simulink model "CAMFC2_04_Quad_03_R2017b"  (R2017b)
settings: Solver=ode45  StartTime=0.0  StopTime=600  RelTol=1e-3  EnableMultiTasking=on
InitFcn:
  | constant_CAMFC2_04_Quad_03
values from neighbouring files (symbols this model uses):
  alpha = 0.1    [constant_CAMFC2_01_WMR01.m]    (also in constant_CAMFC2_04_Comp.m = 0.01; constant_CAMFC2_04_Quad_03.m; constant_CAMFC2_04_Simple.m = 0.01; constant_CAMFC2_04_Simple_DoubleIntegrator.m = 0.01)
  AN = [     0 1 0 0 ... (first row only)    [constant_CAMFC2_01_WMR01.m]    (also in constant_CAMFC2_04_Comp.m = [     0 1 0 0 1; constant_CAMFC2_04_Quad_03.m; constant_CAMFC2_04_Simple.m; constant_CAMFC2_04_Simple_DoubleIntegrator.m)
  B = eye(n)    [constant_CAMFC2_01_WMR01.m]    (also in constant_CAMFC2_04_Quad_03.m; constant_CAMFC2_Quad_New_02.m)
  BBT_inv = ((B'*B)^(-1))*B'    [constant_CAMFC2_04_Quad_03.m]    (also in constant_CAMFC2_Quad_New_02.m)
  Beta = 0.2    [constant_CAMFC2_04_Quad_03.m]    (also in constant_CAMFC2_Quad_New_02.m = 0.1)
  BN = [     1 0 0 0 ... (first row only)    [constant_CAMFC2_01_WMR01.m]    (also in constant_CAMFC2_04_Comp.m = [     0 0 0 0 0; constant_CAMFC2_04_Quad_03.m; constant_CAMFC2_04_Simple.m; constant_CAMFC2_04_Simple_DoubleIntegrator.m)
  Bv = eye(n0)    [constant_CAMFC2_04_Quad_03.m]
  BvBT_inv = ((Bv'*Bv)^(-1))*Bv'    [constant_CAMFC2_04_Quad_03.m]
  chi = [0 0 0 0 ... (first row only)    [constant_CAMFC2_01_WMR01.m]    (also in constant_CAMFC2_04_Comp.m = X_m*ones(n0,1); constant_CAMFC2_04_Quad_03.m = X_m*ones(n0,1); constant_CAMFC2_04_Simple.m = X_m*ones(n0,1); constant_CAMFC2_04_Simple_DoubleIntegrator.m = X_m*ones(n0,1))
  epsilon_struct = struct('data',epsilon_InitVal)    [constant_CAMFC2_01_WMR01.m]    (also in constant_CAMFC2_04_Comp.m; constant_CAMFC2_04_Quad_03.m; constant_CAMFC2_04_Simple.m; constant_CAMFC2_04_Simple_DoubleIntegrator.m)
  gama1 = 1e4*diag([1e-6*ones(2,1);1e0*ones(2,1)])    [constant_CAMFC2_01_WMR01.m]    (also in constant_CAMFC2_04_Comp.m = 1e+3*diag([1e-6;1e-0]); constant_CAMFC2_04_Quad_03.m = 1e+2*diag(1e-0*ones(n0,1)); constant_CAMFC2_04_Simple.m = 1e+2*diag([1e-0;1e-0]); constant_CAMFC2_04_Simple_Formation.m = 1e+2*diag([1e-0;1e-0]))
  gama2 = 1e-2*diag([1e-6*ones(2,1);1e0*ones(2,1)])    [constant_CAMFC2_01_WMR01.m]    (also in constant_CAMFC2_04_Comp.m = 1e+0*diag([1e-6;1e-0]); constant_CAMFC2_04_Quad_03.m = 1e+0*diag(1e-0*ones(n0,1)); constant_CAMFC2_04_Simple.m = 1e+1*diag([1e-0;1e-0]); constant_CAMFC2_04_Simple_Formation.m = 1e+1*diag([1e-0;1e-0]))
  gamma_0 = 1e+0*diag([1e-0*ones(n0,1);1e-0*ones(n0,1)])    [constant_CAMFC2_04_Quad_03.m]    (also in constant_CAMFC2_Quad_New_02.m = 1e-2*diag([1e-6*ones(n0,1);1e-0*ones(n0,1)]))
  gamma_0v = 1e-0*diag(1e-0*ones(n0,1))    [constant_CAMFC2_04_Quad_03.m]
  gamma_1 = 1e+2*diag([1e-0*ones(n0,1);1e-0*ones(n0,1)])    [constant_CAMFC2_04_Quad_03.m]    (also in constant_CAMFC2_Quad_New_02.m = 1e+1*diag([1e-6*ones(n0,1);1e-0*ones(n0,1)]))
  gamma_1v = 1e+2*diag(1e-0*ones(n0,1))    [constant_CAMFC2_04_Quad_03.m]
  ge = 9.81    [constant_CAMFC2_04_Comp.m]    (also in constant_CAMFC2_04_Quad_03.m; constant_CAMFC2_04_Simple.m; constant_CAMFC2_04_Simple_DoubleIntegrator.m; constant_CAMFC2_04_Simple_DoubleIntegrator_02.m)
  H = L + BN    [constant_CAMFC2_01_WMR01.m]    (also in constant_CAMFC2_04_Comp.m; constant_CAMFC2_04_Quad_03.m; constant_CAMFC2_04_Simple.m; constant_CAMFC2_04_Simple_DoubleIntegrator.m)
  J = 0.01    [constant_CAMFC2_01_WMR01.m]    (also in constant_CAMFC2_04_Quad_03.m = 1.0e-3 * diag([1 1 2],0); constant_CAMFC2_Quad_New_02.m = 1.2416e-3 * diag([1 1 2],0))
  k1 = 1    [constant_CAMFC2_01_WMR01.m]    (also in constant_CAMFC2_04_Comp.m; constant_CAMFC2_04_Quad_03.m = 50; constant_CAMFC2_04_Simple.m; constant_CAMFC2_04_Simple_DoubleIntegrator.m)
  k2 = 1    [constant_CAMFC2_01_WMR01.m]    (also in constant_CAMFC2_04_Comp.m; constant_CAMFC2_04_Quad_03.m; constant_CAMFC2_04_Simple.m; constant_CAMFC2_04_Simple_DoubleIntegrator.m)
  Ka = 0.1    [constant_CAMFC2_04_Quad_03.m]    (also in constant_CAMFC2_Quad_New_02.m = 0.01)
  Kd = 0.1    [constant_CAMFC2_04_Quad_03.m]    (also in constant_CAMFC2_Quad_New_02.m = 0.01)
  m = 6    [constant_CAMFC2_04_Quad_03.m]    (also in constant_CAMFC2_Quad_New_02.m)
  M = 1    [constant_CAMFC2_01_WMR01.m]    (also in constant_CAMFC2_04_Quad_03.m = 2; constant_CAMFC2_Quad_New_02.m = 2)
  N = 4    [constant_CAMFC2_01_WMR01.m]    (also in constant_CAMFC2_04_Comp.m = 5; constant_CAMFC2_04_Quad_03.m; constant_CAMFC2_04_Simple.m; constant_CAMFC2_04_Simple_DoubleIntegrator.m)
  n = 4    [constant_CAMFC2_01_WMR01.m]    (also in constant_CAMFC2_04_Comp.m = 2; constant_CAMFC2_04_Quad_03.m = 6; constant_CAMFC2_04_Simple.m = 2; constant_CAMFC2_04_Simple_DoubleIntegrator.m = 2)
  n0 = 2    [constant_CAMFC2_01_WMR01.m]    (also in constant_CAMFC2_04_Comp.m = 1; constant_CAMFC2_04_Quad_03.m = 3; constant_CAMFC2_04_Simple.m; constant_CAMFC2_04_Simple_DoubleIntegrator.m = 1)
  noise_amp = 0.1    [constant_CAMFC2_04_Quad_03.m]
  noise_frq = 1    [constant_CAMFC2_04_Quad_03.m]
  Observer_Gain = 100    [constant_CAMFC2_01_WMR01.m]    (also in constant_CAMFC2_04_Comp.m = 10; constant_CAMFC2_04_Quad_03.m = 1; constant_CAMFC2_04_Simple.m; constant_CAMFC2_04_Simple_DoubleIntegrator.m)
  Observer_Gain1 = 100    [constant_CAMFC2_01_WMR01.m]    (also in constant_CAMFC2_04_Comp.m = 10; constant_CAMFC2_04_Quad_03.m = 1; constant_CAMFC2_04_Simple.m; constant_CAMFC2_04_Simple_DoubleIntegrator.m)
  P_struct = struct('data',P_InitVal)    [constant_CAMFC2_01_WMR01.m]    (also in constant_CAMFC2_04_Comp.m; constant_CAMFC2_04_Quad_03.m; constant_CAMFC2_04_Simple.m; constant_CAMFC2_04_Simple_DoubleIntegrator.m)
  Q = 1e-0*eye(n)    [constant_CAMFC2_01_WMR01.m]    (also in constant_CAMFC2_04_Comp.m = 1.0e+2*eye(n); constant_CAMFC2_04_Quad_03.m = 1e-0*eye(n0); constant_CAMFC2_04_Simple.m = 1.0e+1*eye(n); constant_CAMFC2_04_Simple_Formation.m = 1.0e+1*eye(n))
  QR = 1e-0*eye(n)    [constant_CAMFC2_04_Quad_03.m]    (also in constant_CAMFC2_Quad_New_02.m = 1e+0*eye(n))
  Qv = 1e-0*eye(n0)    [constant_CAMFC2_04_Quad_03.m]
  R = 1e-0*eye(n)    [constant_CAMFC2_01_WMR01.m]    (also in constant_CAMFC2_04_Quad_03.m; constant_CAMFC2_Quad_New_02.m = 1e+0*eye(n))
  r_formX = 1.0    (= 1)    [constant_CAMFC2_04_Quad_03.m]    (also in constant_CAMFC2_Quad_New_02.m)
  r_formY = 1.0    (= 1)    [constant_CAMFC2_04_Quad_03.m]    (also in constant_CAMFC2_Quad_New_02.m)
  r_formZ = 0.5    [constant_CAMFC2_04_Quad_03.m]    (also in constant_CAMFC2_Quad_New_02.m = 1)
  rho1 = 1e-1    (= 0.1)    [constant_CAMFC2_01_WMR01.m]    (also in constant_CAMFC2_04_Comp.m = 1; constant_CAMFC2_04_Quad_03.m = 1; constant_CAMFC2_04_Simple.m = 1; constant_CAMFC2_04_Simple_DoubleIntegrator.m = 1)
  rho2 = 1e-3    (= 0.001)    [constant_CAMFC2_01_WMR01.m]    (also in constant_CAMFC2_04_Comp.m = 1; constant_CAMFC2_04_Quad_03.m = 1; constant_CAMFC2_04_Simple.m = 1; constant_CAMFC2_04_Simple_DoubleIntegrator.m = 10)
  rho_0 = 1e-0    (= 1)    [constant_CAMFC2_04_Quad_03.m]    (also in constant_CAMFC2_Quad_New_02.m = 0.01)
  rho_0v = 1e-0    (= 1)    [constant_CAMFC2_04_Quad_03.m]
  rho_1 = 1e-0    (= 1)    [constant_CAMFC2_04_Quad_03.m]    (also in constant_CAMFC2_Quad_New_02.m = 0.01)
  rho_1v = 1e-0    (= 1)    [constant_CAMFC2_04_Quad_03.m]
  Rv = 1e-0*eye(n0)    [constant_CAMFC2_04_Quad_03.m]
  T_struct = struct('data',T_InitVal)    [constant_CAMFC2_01_WMR01.m]    (also in constant_CAMFC2_04_Comp.m; constant_CAMFC2_04_Quad_03.m; constant_CAMFC2_04_Simple.m; constant_CAMFC2_04_Simple_DoubleIntegrator.m)
  Upsilon_M = Upsilon_m*ones(n,1)    [constant_CAMFC2_01_WMR01.m]    (also in constant_CAMFC2_04_Comp.m; constant_CAMFC2_04_Quad_03.m = Upsilon_m*ones(n0,1); constant_CAMFC2_04_Simple.m; constant_CAMFC2_04_Simple_DoubleIntegrator.m)
  Vel_limit = 100    [constant_CAMFC2_04_Quad_03.m]
(part 2 of 4)

== system CAMFC2_04_Quad_03_R2017b/Data Bus /Observers Log/For matrix Plot11 ==
  T : Inport
  MATLAB Function : MATLAB Function  TreatAsAtomicUnit=on
  To Workspace : ToWorkspace  VariableName=T4  SaveFormat=Structure With Time  SampleTime=-1
  wires:
  MATLAB Function/1(y) -> To Workspace/1
  T/1 -> MATLAB Function/1(u)

== system CAMFC2_04_Quad_03_R2017b/Data Bus /Observers Log/For matrix Plot12 ==
  epsilon : Inport
  MATLAB Function : MATLAB Function  TreatAsAtomicUnit=on
  To Workspace : ToWorkspace  VariableName=epsilon1  SaveFormat=Structure With Time  SampleTime=-1
  wires:
  epsilon/1 -> MATLAB Function/1(u)
  MATLAB Function/1(y) -> To Workspace/1

== system CAMFC2_04_Quad_03_R2017b/Data Bus /Observers Log/For matrix Plot13 ==
  epsilon : Inport
  MATLAB Function : MATLAB Function  TreatAsAtomicUnit=on
  To Workspace : ToWorkspace  VariableName=epsilon2  SaveFormat=Structure With Time  SampleTime=-1
  wires:
  MATLAB Function/1(y) -> To Workspace/1
  epsilon/1 -> MATLAB Function/1(u)

== system CAMFC2_04_Quad_03_R2017b/Data Bus /Observers Log/For matrix Plot14 ==
  epsilon : Inport
  MATLAB Function : MATLAB Function  TreatAsAtomicUnit=on
  To Workspace : ToWorkspace  VariableName=epsilon3  SaveFormat=Structure With Time  SampleTime=-1
  wires:
  MATLAB Function/1(y) -> To Workspace/1
  epsilon/1 -> MATLAB Function/1(u)

== system CAMFC2_04_Quad_03_R2017b/Data Bus /Observers Log/For matrix Plot15 ==
  epsilon : Inport
  MATLAB Function : MATLAB Function  TreatAsAtomicUnit=on
  To Workspace : ToWorkspace  VariableName=epsilon4  SaveFormat=Structure With Time  SampleTime=-1
  wires:
  epsilon/1 -> MATLAB Function/1(u)
  MATLAB Function/1(y) -> To Workspace/1

== system CAMFC2_04_Quad_03_R2017b/Data Bus /Observers Log/For matrix Plot8 ==
  T : Inport
  MATLAB Function : MATLAB Function  TreatAsAtomicUnit=on
  To Workspace : ToWorkspace  VariableName=T1  SaveFormat=Structure With Time  SampleTime=-1
  wires:
  MATLAB Function/1(y) -> To Workspace/1
  T/1 -> MATLAB Function/1(u)

== system CAMFC2_04_Quad_03_R2017b/Data Bus /Observers Log/For matrix Plot9 ==
  T : Inport
  MATLAB Function : MATLAB Function  TreatAsAtomicUnit=on
  To Workspace : ToWorkspace  VariableName=T2  SaveFormat=Structure With Time  SampleTime=-1
  wires:
  T/1 -> MATLAB Function/1(u)
  MATLAB Function/1(y) -> To Workspace/1

== system CAMFC2_04_Quad_03_R2017b/Data Bus /Reference Trajectory/Subsystem ==
  Clock1 : Clock
  Desired Position4 : Constant  Value=0  VectorParams1D=off
  From Workspace : FromWorkspace  VariableName=RECT_X  SampleTime=0
  From Workspace1 : FromWorkspace  VariableName=RECT_Y  SampleTime=0
  From Workspace3 : FromWorkspace  VariableName=RECT_Z  SampleTime=0
  Gain : Gain  Gain=1/5
  Gain1 : Gain  Gain=1/5
  Gain2 : Gain
  Scope2 : Scope  NumInputPorts=3
  Switch : Switch  Criteria=u2 > Threshold  Threshold=10
  Transfer Fcn1 : TransferFcn  Numerator=[Beta]  Denominator=[1 Beta]
  Transfer Fcn2 : TransferFcn  Numerator=[Beta]  Denominator=[1 Beta]
  Transfer Fcn3 : TransferFcn  Numerator=[Beta]  Denominator=[1 Beta]
  Xd : Outport
  Yd : Outport  Port=2
  Zd : Outport  Port=3
  wires:
  From Workspace/1 -> Gain/1
  From Workspace1/1 -> Gain1/1
  Clock1/1 -> Switch/2
  Switch/1 -> Transfer Fcn1/1
  From Workspace3/1 -> Gain2/1
  Desired Position4/1 -> Switch/3
  Transfer Fcn1/1 -> Zd/1, Scope2/3
  Transfer Fcn2/1 -> Yd/1, Scope2/2
  Transfer Fcn3/1 -> Xd/1, Scope2/1
  Gain/1 -> Transfer Fcn3/1
  Gain1/1 -> Transfer Fcn2/1
  Gain2/1 -> Switch/1

== system CAMFC2_04_Quad_03_R2017b/Data Bus /Rotational Log/For matrix Plot ==
  P : Inport
  MATLAB Function : MATLAB Function  TreatAsAtomicUnit=on
  To Workspace : ToWorkspace  VariableName=P1_R  SaveFormat=Structure With Time  SampleTime=-1
  wires:
  MATLAB Function/1(y) -> To Workspace/1
  P/1 -> MATLAB Function/1(u)

== system CAMFC2_04_Quad_03_R2017b/Data Bus /Rotational Log/For matrix Plot1 ==
  P : Inport
  MATLAB Function : MATLAB Function  TreatAsAtomicUnit=on
  To Workspace : ToWorkspace  VariableName=P2_R  SaveFormat=Structure With Time  SampleTime=-1
  wires:
  P/1 -> MATLAB Function/1(u)
  MATLAB Function/1(y) -> To Workspace/1

== system CAMFC2_04_Quad_03_R2017b/Data Bus /Rotational Log/For matrix Plot2 ==
  P : Inport
  MATLAB Function : MATLAB Function  TreatAsAtomicUnit=on
  To Workspace : ToWorkspace  VariableName=P3_R  SaveFormat=Structure With Time  SampleTime=-1
  wires:
  P/1 -> MATLAB Function/1(u)
  MATLAB Function/1(y) -> To Workspace/1

== system CAMFC2_04_Quad_03_R2017b/Data Bus /Rotational Log/For matrix Plot3 ==
  P : Inport
  MATLAB Function : MATLAB Function  TreatAsAtomicUnit=on
  To Workspace : ToWorkspace  VariableName=P4_R  SaveFormat=Structure With Time  SampleTime=-1
  wires:
  MATLAB Function/1(y) -> To Workspace/1
  P/1 -> MATLAB Function/1(u)

== system CAMFC2_04_Quad_03_R2017b/Data Bus /Rotational Log/For matrix Plot4 ==
  A_hat : Inport
  MATLAB Function : MATLAB Function  TreatAsAtomicUnit=on
  To Workspace : ToWorkspace  VariableName=A_hat1_R  SaveFormat=Structure With Time  SampleTime=-1
  wires:
  A_hat/1 -> MATLAB Function/1(u)
  MATLAB Function/1(y) -> To Workspace/1

== system CAMFC2_04_Quad_03_R2017b/Data Bus /Rotational Log/For matrix Plot5 ==
  A_hat : Inport
  MATLAB Function : MATLAB Function  TreatAsAtomicUnit=on
  To Workspace : ToWorkspace  VariableName=A_hat2_R  SaveFormat=Structure With Time  SampleTime=-1
  wires:
  MATLAB Function/1(y) -> To Workspace/1
  A_hat/1 -> MATLAB Function/1(u)

== system CAMFC2_04_Quad_03_R2017b/Data Bus /Rotational Log/For matrix Plot6 ==
  A_hat : Inport
  MATLAB Function : MATLAB Function  TreatAsAtomicUnit=on
  To Workspace : ToWorkspace  VariableName=A_hat3_R  SaveFormat=Structure With Time  SampleTime=-1
  wires:
  A_hat/1 -> MATLAB Function/1(u)
  MATLAB Function/1(y) -> To Workspace/1

== system CAMFC2_04_Quad_03_R2017b/Data Bus /Rotational Log/For matrix Plot7 ==
  A_hat : Inport
  MATLAB Function : MATLAB Function  TreatAsAtomicUnit=on
  To Workspace : ToWorkspace  VariableName=A_hat4_R  SaveFormat=Structure With Time  SampleTime=-1
  wires:
  MATLAB Function/1(y) -> To Workspace/1
  A_hat/1 -> MATLAB Function/1(u)

== system CAMFC2_04_Quad_03_R2017b/Data Bus /Translational Log/For matrix Plot ==
  P : Inport
  MATLAB Function : MATLAB Function  TreatAsAtomicUnit=on
  To Workspace : ToWorkspace  VariableName=P1_TP  SaveFormat=Structure With Time  SampleTime=-1
  wires:
  P/1 -> MATLAB Function/1(u)
  MATLAB Function/1(y) -> To Workspace/1

== system CAMFC2_04_Quad_03_R2017b/Data Bus /Translational Log/For matrix Plot1 ==
  P : Inport
  MATLAB Function : MATLAB Function  TreatAsAtomicUnit=on
  To Workspace : ToWorkspace  VariableName=P2_TP  SaveFormat=Structure With Time  SampleTime=-1
  wires:
  MATLAB Function/1(y) -> To Workspace/1
  P/1 -> MATLAB Function/1(u)

== system CAMFC2_04_Quad_03_R2017b/Data Bus /Translational Log/For matrix Plot2 ==
  P : Inport
  MATLAB Function : MATLAB Function  TreatAsAtomicUnit=on
  To Workspace : ToWorkspace  VariableName=P3_TP  SaveFormat=Structure With Time  SampleTime=-1
  wires:
  MATLAB Function/1(y) -> To Workspace/1
  P/1 -> MATLAB Function/1(u)

== system CAMFC2_04_Quad_03_R2017b/Data Bus /Translational Log/For matrix Plot3 ==
  P : Inport
  MATLAB Function : MATLAB Function  TreatAsAtomicUnit=on
  To Workspace : ToWorkspace  VariableName=P4_TP  SaveFormat=Structure With Time  SampleTime=-1
  wires:
  P/1 -> MATLAB Function/1(u)
  MATLAB Function/1(y) -> To Workspace/1

== system CAMFC2_04_Quad_03_R2017b/Data Bus /Translational Log/For matrix Plot4 ==
  A_hat : Inport
  MATLAB Function : MATLAB Function  TreatAsAtomicUnit=on
  To Workspace : ToWorkspace  VariableName=A_hat1_TP  SaveFormat=Structure With Time  SampleTime=-1
  wires:
  MATLAB Function/1(y) -> To Workspace/1
  A_hat/1 -> MATLAB Function/1(u)

== system CAMFC2_04_Quad_03_R2017b/Data Bus /Translational Log/For matrix Plot5 ==
  A_hat : Inport
  MATLAB Function : MATLAB Function  TreatAsAtomicUnit=on
  To Workspace : ToWorkspace  VariableName=A_hat2_TP  SaveFormat=Structure With Time  SampleTime=-1
  wires:
  A_hat/1 -> MATLAB Function/1(u)
  MATLAB Function/1(y) -> To Workspace/1

== system CAMFC2_04_Quad_03_R2017b/Data Bus /Translational Log/For matrix Plot6 ==
  A_hat : Inport
  MATLAB Function : MATLAB Function  TreatAsAtomicUnit=on
  To Workspace : ToWorkspace  VariableName=A_hat3_TP  SaveFormat=Structure With Time  SampleTime=-1
  wires:
  MATLAB Function/1(y) -> To Workspace/1
  A_hat/1 -> MATLAB Function/1(u)

== system CAMFC2_04_Quad_03_R2017b/Data Bus /Translational Log/For matrix Plot7 ==
  A_hat : Inport
  MATLAB Function : MATLAB Function  TreatAsAtomicUnit=on
  To Workspace : ToWorkspace  VariableName=A_hat4_TP  SaveFormat=Structure With Time  SampleTime=-1
  wires:
  A_hat/1 -> MATLAB Function/1(u)
  MATLAB Function/1(y) -> To Workspace/1

== system CAMFC2_04_Quad_03_R2017b/Data Bus /Velocity Log/For matrix Plot ==
  P : Inport
  MATLAB Function : MATLAB Function  TreatAsAtomicUnit=on
  To Workspace : ToWorkspace  VariableName=P1_V  SaveFormat=Structure With Time  SampleTime=-1
  wires:
  P/1 -> MATLAB Function/1(u)
  MATLAB Function/1(y) -> To Workspace/1

== system CAMFC2_04_Quad_03_R2017b/Data Bus /Velocity Log/For matrix Plot1 ==
  P : Inport
  MATLAB Function : MATLAB Function  TreatAsAtomicUnit=on
  To Workspace : ToWorkspace  VariableName=P2_V  SaveFormat=Structure With Time  SampleTime=-1
  wires:
  MATLAB Function/1(y) -> To Workspace/1
  P/1 -> MATLAB Function/1(u)

== system CAMFC2_04_Quad_03_R2017b/Data Bus /Velocity Log/For matrix Plot2 ==
  P : Inport
  MATLAB Function : MATLAB Function  TreatAsAtomicUnit=on
  To Workspace : ToWorkspace  VariableName=P3_V  SaveFormat=Structure With Time  SampleTime=-1
  wires:
  MATLAB Function/1(y) -> To Workspace/1
  P/1 -> MATLAB Function/1(u)

== system CAMFC2_04_Quad_03_R2017b/Data Bus /Velocity Log/For matrix Plot3 ==
  P : Inport
  MATLAB Function : MATLAB Function  TreatAsAtomicUnit=on
  To Workspace : ToWorkspace  VariableName=P4_V  SaveFormat=Structure With Time  SampleTime=-1
  wires:
  P/1 -> MATLAB Function/1(u)
  MATLAB Function/1(y) -> To Workspace/1

== system CAMFC2_04_Quad_03_R2017b/Data Bus /Velocity Log/For matrix Plot4 ==
  A_hat : Inport
  MATLAB Function : MATLAB Function  TreatAsAtomicUnit=on
  To Workspace : ToWorkspace  VariableName=A_hat1_V  SaveFormat=Structure With Time  SampleTime=-1
  wires:
  MATLAB Function/1(y) -> To Workspace/1
  A_hat/1 -> MATLAB Function/1(u)

== system CAMFC2_04_Quad_03_R2017b/Data Bus /Velocity Log/For matrix Plot5 ==
  A_hat : Inport
  MATLAB Function : MATLAB Function  TreatAsAtomicUnit=on
  To Workspace : ToWorkspace  VariableName=A_hat2_V  SaveFormat=Structure With Time  SampleTime=-1
  wires:
  A_hat/1 -> MATLAB Function/1(u)
  MATLAB Function/1(y) -> To Workspace/1

== system CAMFC2_04_Quad_03_R2017b/Data Bus /Velocity Log/For matrix Plot6 ==
  A_hat : Inport
  MATLAB Function : MATLAB Function  TreatAsAtomicUnit=on
  To Workspace : ToWorkspace  VariableName=A_hat3_V  SaveFormat=Structure With Time  SampleTime=-1
  wires:
  MATLAB Function/1(y) -> To Workspace/1
  A_hat/1 -> MATLAB Function/1(u)

== system CAMFC2_04_Quad_03_R2017b/Data Bus /Velocity Log/For matrix Plot7 ==
  A_hat : Inport
  MATLAB Function : MATLAB Function  TreatAsAtomicUnit=on
  To Workspace : ToWorkspace  VariableName=A_hat4_V  SaveFormat=Structure With Time  SampleTime=-1
  wires:
  A_hat/1 -> MATLAB Function/1(u)
  MATLAB Function/1(y) -> To Workspace/1

== system CAMFC2_04_Quad_03_R2017b/Agent #1/Decenteralized Cooperaive Controller #1/Cooperative Position Controller #1/DRE1 ==
  Agent_Num : Inport
  A_hat : Inport  Port=2
  Demux : Demux  Outputs=3
  MATLAB Function : MATLAB Function  TreatAsAtomicUnit=on
  MATLAB Function1 : MATLAB Function  TreatAsAtomicUnit=on
  Mux : Mux  Inputs=3
  P1 : Subsystem
  P2 : Subsystem
  P3 : Subsystem
  P : Outport
  wires:
  Demux/1 -> P1/1(a1)
  Agent_Num/1 -> P1/2(Agent_Num), P2/2(Agent_Num), P3/2(Agent_Num)
  A_hat/1 -> MATLAB Function/1(inp)
  MATLAB Function/1(otp) -> Demux/1
  P1/1(p1) -> Mux/1
  Mux/1 -> MATLAB Function1/1(inp)
  MATLAB Function1/1(otp) -> P/1
  Demux/2 -> P2/1(a2)
  Demux/3 -> P3/1(a3)
  P2/1(p2) -> Mux/2
  P3/1(p3) -> Mux/3

== system CAMFC2_04_Quad_03_R2017b/Agent #1/Decenteralized Cooperaive Controller #1/Cooperative Position Controller #1/Differentiator0 ==
  x_d : Inport
  Integrator : Integrator  InitialCondition=zeros(n0,1)
  Integrator1 : Integrator  InitialCondition=zeros(n0,1)
  Sliding differentiator : MATLAB Function  TreatAsAtomicUnit=on
  Sliding differentiator1 : MATLAB Function  TreatAsAtomicUnit=on
  Sum : Sum  Inputs=|-+
  Dx_d : Outport
  wires:
  Sliding differentiator/1(u) -> Integrator1/1, Dx_d/1
  Sliding differentiator1/1(Du1) -> Integrator/1
  Integrator/1 -> Sliding differentiator/1(u1)
  x_d/1 -> Sum/1
  Sum/1 -> Sliding differentiator/2(e), Sliding differentiator1/1(e)
  Integrator1/1 -> Sum/2

== system CAMFC2_04_Quad_03_R2017b/Agent #1/Decenteralized Cooperaive Controller #1/Cooperative Position Controller #1/Differentiator2 ==
  x_d : Inport
  Integrator : Integrator  InitialCondition=zeros(N+1,n0)
  Integrator1 : Integrator  InitialCondition=zeros(N+1,n0)
  Sliding differentiator : MATLAB Function  TreatAsAtomicUnit=on
  Sliding differentiator1 : MATLAB Function  TreatAsAtomicUnit=on
  Sum : Sum  Inputs=|-+
  Dx_d : Outport
  wires:
  Sliding differentiator/1(u) -> Integrator1/1, Dx_d/1
  Sliding differentiator1/1(Du1) -> Integrator/1
  Integrator/1 -> Sliding differentiator/1(u1)
  x_d/1 -> Sum/1
  Sum/1 -> Sliding differentiator/2(e), Sliding differentiator1/1(e)
  Integrator1/1 -> Sum/2

== system CAMFC2_04_Quad_03_R2017b/Agent #1/Decenteralized Cooperaive Controller #1/Rotational AMFC #1/Differentiator ==
  x_d : Inport
  Integrator : Integrator  InitialCondition=zeros(n,1)
  Integrator1 : Integrator  InitialCondition=zeros(n,1)
  Sliding differentiator : MATLAB Function  TreatAsAtomicUnit=on
  Sliding differentiator1 : MATLAB Function  TreatAsAtomicUnit=on
  Sum : Sum  Inputs=|-+
  Dx_d : Outport
  wires:
  Sliding differentiator/1(u) -> Integrator1/1, Dx_d/1
  Sliding differentiator1/1(Du1) -> Integrator/1
  Integrator/1 -> Sliding differentiator/1(u1)
  x_d/1 -> Sum/1
  Sum/1 -> Sliding differentiator/2(e), Sliding differentiator1/1(e)
  Integrator1/1 -> Sum/2

== system CAMFC2_04_Quad_03_R2017b/Agent #1/Decenteralized Cooperaive Controller #1/Velocity AMFC #1/Differentiator ==
  x_d : Inport
  Integrator : Integrator  InitialCondition=zeros(n0,1)
  Integrator1 : Integrator  InitialCondition=zeros(n0,1)
  Sliding differentiator : MATLAB Function  TreatAsAtomicUnit=on
  Sliding differentiator1 : MATLAB Function  TreatAsAtomicUnit=on
  Sum : Sum  Inputs=|-+
  Dx_d : Outport
  wires:
  Sliding differentiator/1(u) -> Integrator1/1, Dx_d/1
  Sliding differentiator1/1(Du1) -> Integrator/1
  Integrator/1 -> Sliding differentiator/1(u1)
  x_d/1 -> Sum/1
  Sum/1 -> Sliding differentiator/2(e), Sliding differentiator1/1(e)
  Integrator1/1 -> Sum/2

== system CAMFC2_04_Quad_03_R2017b/Agent #2/Decenteralized Cooperaive Controller #2/Cooperative Position Controller #2/DRE2 ==
  Agent_Num : Inport
  A_hat : Inport  Port=2
  Demux : Demux  Outputs=3
  MATLAB Function : MATLAB Function  TreatAsAtomicUnit=on
  MATLAB Function1 : MATLAB Function  TreatAsAtomicUnit=on
  Mux : Mux  Inputs=3
  P1 : Subsystem
  P2 : Subsystem
  P3 : Subsystem
  P : Outport
  wires:
  P3/1(p3) -> Mux/3
  P2/1(p2) -> Mux/2
  Demux/3 -> P3/1(a3)
  Demux/2 -> P2/1(a2)
  MATLAB Function1/1(otp) -> P/1
  Mux/1 -> MATLAB Function1/1(inp)
  P1/1(p1) -> Mux/1
  MATLAB Function/1(otp) -> Demux/1
  A_hat/1 -> MATLAB Function/1(inp)
  Agent_Num/1 -> P3/2(Agent_Num), P2/2(Agent_Num), P1/2(Agent_Num)
  Demux/1 -> P1/1(a1)

== system CAMFC2_04_Quad_03_R2017b/Agent #2/Decenteralized Cooperaive Controller #2/Cooperative Position Controller #2/Differentiator0 ==
  x_d : Inport
  Integrator : Integrator  InitialCondition=zeros(n0,1)
  Integrator1 : Integrator  InitialCondition=zeros(n0,1)
  Sliding differentiator : MATLAB Function  TreatAsAtomicUnit=on
  Sliding differentiator1 : MATLAB Function  TreatAsAtomicUnit=on
  Sum : Sum  Inputs=|-+
  Dx_d : Outport
  wires:
  Sliding differentiator/1(u) -> Integrator1/1, Dx_d/1
  Sliding differentiator1/1(Du1) -> Integrator/1
  Integrator/1 -> Sliding differentiator/1(u1)
  x_d/1 -> Sum/1
  Sum/1 -> Sliding differentiator/2(e), Sliding differentiator1/1(e)
  Integrator1/1 -> Sum/2

== system CAMFC2_04_Quad_03_R2017b/Agent #2/Decenteralized Cooperaive Controller #2/Cooperative Position Controller #2/Differentiator2 ==
  x_d : Inport
  Integrator : Integrator  InitialCondition=zeros(N+1,n0)
  Integrator1 : Integrator  InitialCondition=zeros(N+1,n0)
  Sliding differentiator : MATLAB Function  TreatAsAtomicUnit=on
  Sliding differentiator1 : MATLAB Function  TreatAsAtomicUnit=on
  Sum : Sum  Inputs=|-+
  Dx_d : Outport
  wires:
  Integrator1/1 -> Sum/2
  Sum/1 -> Sliding differentiator1/1(e), Sliding differentiator/2(e)
  x_d/1 -> Sum/1
  Integrator/1 -> Sliding differentiator/1(u1)
  Sliding differentiator1/1(Du1) -> Integrator/1
  Sliding differentiator/1(u) -> Dx_d/1, Integrator1/1

== system CAMFC2_04_Quad_03_R2017b/Agent #2/Decenteralized Cooperaive Controller #2/Rotational AMFC #2/Differentiator ==
  x_d : Inport
  Integrator : Integrator  InitialCondition=zeros(n,1)
  Integrator1 : Integrator  InitialCondition=zeros(n,1)
  Sliding differentiator : MATLAB Function  TreatAsAtomicUnit=on
  Sliding differentiator1 : MATLAB Function  TreatAsAtomicUnit=on
  Sum : Sum  Inputs=|-+
  Dx_d : Outport
  wires:
  Integrator1/1 -> Sum/2
  Sum/1 -> Sliding differentiator1/1(e), Sliding differentiator/2(e)
  x_d/1 -> Sum/1
  Integrator/1 -> Sliding differentiator/1(u1)
  Sliding differentiator1/1(Du1) -> Integrator/1
  Sliding differentiator/1(u) -> Dx_d/1, Integrator1/1

== system CAMFC2_04_Quad_03_R2017b/Agent #2/Decenteralized Cooperaive Controller #2/Velocity AMFC #2/Differentiator ==
  x_d : Inport
  Integrator : Integrator  InitialCondition=zeros(n0,1)
  Integrator1 : Integrator  InitialCondition=zeros(n0,1)
  Sliding differentiator : MATLAB Function  TreatAsAtomicUnit=on
  Sliding differentiator1 : MATLAB Function  TreatAsAtomicUnit=on
  Sum : Sum  Inputs=|-+
  Dx_d : Outport
  wires:
  Integrator1/1 -> Sum/2
  Sum/1 -> Sliding differentiator1/1(e), Sliding differentiator/2(e)
  x_d/1 -> Sum/1
  Integrator/1 -> Sliding differentiator/1(u1)
  Sliding differentiator1/1(Du1) -> Integrator/1
  Sliding differentiator/1(u) -> Dx_d/1, Integrator1/1

== system CAMFC2_04_Quad_03_R2017b/Agent #3/Decenteralized Cooperaive Controller #3/Cooperative Position Controller #3/DRE3 ==
  Agent_Num : Inport
  A_hat : Inport  Port=2
  Demux : Demux  Outputs=3
  MATLAB Function : MATLAB Function  TreatAsAtomicUnit=on
  MATLAB Function1 : MATLAB Function  TreatAsAtomicUnit=on
  Mux : Mux  Inputs=3
  P1 : Subsystem
  P2 : Subsystem
  P3 : Subsystem
  P : Outport
  wires:
  Demux/1 -> P1/1(a1)
  Agent_Num/1 -> P1/2(Agent_Num), P2/2(Agent_Num), P3/2(Agent_Num)
  A_hat/1 -> MATLAB Function/1(inp)
  MATLAB Function/1(otp) -> Demux/1
  P1/1(p1) -> Mux/1
  Mux/1 -> MATLAB Function1/1(inp)
  MATLAB Function1/1(otp) -> P/1
  Demux/2 -> P2/1(a2)
  Demux/3 -> P3/1(a3)
  P2/1(p2) -> Mux/2
  P3/1(p3) -> Mux/3

== system CAMFC2_04_Quad_03_R2017b/Agent #3/Decenteralized Cooperaive Controller #3/Cooperative Position Controller #3/Differentiator0 ==
  x_d : Inport
  Integrator : Integrator  InitialCondition=zeros(n0,1)
  Integrator1 : Integrator  InitialCondition=zeros(n0,1)
  Sliding differentiator : MATLAB Function  TreatAsAtomicUnit=on
  Sliding differentiator1 : MATLAB Function  TreatAsAtomicUnit=on
  Sum : Sum  Inputs=|-+
  Dx_d : Outport
  wires:
  Sliding differentiator/1(u) -> Integrator1/1, Dx_d/1
  Sliding differentiator1/1(Du1) -> Integrator/1
  Integrator/1 -> Sliding differentiator/1(u1)
  x_d/1 -> Sum/1
  Sum/1 -> Sliding differentiator/2(e), Sliding differentiator1/1(e)
  Integrator1/1 -> Sum/2

== system CAMFC2_04_Quad_03_R2017b/Agent #3/Decenteralized Cooperaive Controller #3/Cooperative Position Controller #3/Differentiator2 ==
  x_d : Inport
  Integrator : Integrator  InitialCondition=zeros(N+1,n0)
  Integrator1 : Integrator  InitialCondition=zeros(N+1,n0)
  Sliding differentiator : MATLAB Function  TreatAsAtomicUnit=on
  Sliding differentiator1 : MATLAB Function  TreatAsAtomicUnit=on
  Sum : Sum  Inputs=|-+
  Dx_d : Outport
  wires:
  Sliding differentiator/1(u) -> Integrator1/1, Dx_d/1
  Sliding differentiator1/1(Du1) -> Integrator/1
  Integrator/1 -> Sliding differentiator/1(u1)
  x_d/1 -> Sum/1
  Sum/1 -> Sliding differentiator/2(e), Sliding differentiator1/1(e)
  Integrator1/1 -> Sum/2

== system CAMFC2_04_Quad_03_R2017b/Agent #3/Decenteralized Cooperaive Controller #3/Rotational AMFC #3/Differentiator ==
  x_d : Inport
  Integrator : Integrator  InitialCondition=zeros(n,1)
  Integrator1 : Integrator  InitialCondition=zeros(n,1)
  Sliding differentiator : MATLAB Function  TreatAsAtomicUnit=on
  Sliding differentiator1 : MATLAB Function  TreatAsAtomicUnit=on
  Sum : Sum  Inputs=|-+
  Dx_d : Outport
  wires:
  Sliding differentiator/1(u) -> Integrator1/1, Dx_d/1
  Sliding differentiator1/1(Du1) -> Integrator/1
  Integrator/1 -> Sliding differentiator/1(u1)
  x_d/1 -> Sum/1
  Sum/1 -> Sliding differentiator/2(e), Sliding differentiator1/1(e)
  Integrator1/1 -> Sum/2

== system CAMFC2_04_Quad_03_R2017b/Agent #3/Decenteralized Cooperaive Controller #3/Velocity AMFC #3/Differentiator ==
  x_d : Inport
  Integrator : Integrator  InitialCondition=zeros(n0,1)
  Integrator1 : Integrator  InitialCondition=zeros(n0,1)
  Sliding differentiator : MATLAB Function  TreatAsAtomicUnit=on
  Sliding differentiator1 : MATLAB Function  TreatAsAtomicUnit=on
  Sum : Sum  Inputs=|-+
  Dx_d : Outport
  wires:
  Sliding differentiator/1(u) -> Integrator1/1, Dx_d/1
  Sliding differentiator1/1(Du1) -> Integrator/1
  Integrator/1 -> Sliding differentiator/1(u1)
  x_d/1 -> Sum/1
  Sum/1 -> Sliding differentiator/2(e), Sliding differentiator1/1(e)
  Integrator1/1 -> Sum/2

== system CAMFC2_04_Quad_03_R2017b/Agent #4/Decenteralized Cooperaive Controller #4/Cooperative Position Controller #4/DRE4 ==
  Agent_Num : Inport
  A_hat : Inport  Port=2
  Demux : Demux  Outputs=3
  MATLAB Function : MATLAB Function  TreatAsAtomicUnit=on
  MATLAB Function1 : MATLAB Function  TreatAsAtomicUnit=on
  Mux : Mux  Inputs=3
  P1 : Subsystem
  P2 : Subsystem
  P3 : Subsystem
  P : Outport
  wires:
  P3/1(p3) -> Mux/3
  P2/1(p2) -> Mux/2
  Demux/3 -> P3/1(a3)
  Demux/2 -> P2/1(a2)
  MATLAB Function1/1(otp) -> P/1
  Mux/1 -> MATLAB Function1/1(inp)
  P1/1(p1) -> Mux/1
  MATLAB Function/1(otp) -> Demux/1
  A_hat/1 -> MATLAB Function/1(inp)
  Agent_Num/1 -> P3/2(Agent_Num), P2/2(Agent_Num), P1/2(Agent_Num)
  Demux/1 -> P1/1(a1)

== system CAMFC2_04_Quad_03_R2017b/Agent #4/Decenteralized Cooperaive Controller #4/Cooperative Position Controller #4/Differentiator0 ==
  x_d : Inport
  Integrator : Integrator  InitialCondition=zeros(n0,1)
  Integrator1 : Integrator  InitialCondition=zeros(n0,1)
  Sliding differentiator : MATLAB Function  TreatAsAtomicUnit=on
  Sliding differentiator1 : MATLAB Function  TreatAsAtomicUnit=on
  Sum : Sum  Inputs=|-+
  Dx_d : Outport
  wires:
  Sliding differentiator/1(u) -> Integrator1/1, Dx_d/1
  Sliding differentiator1/1(Du1) -> Integrator/1
  Integrator/1 -> Sliding differentiator/1(u1)
  x_d/1 -> Sum/1
  Sum/1 -> Sliding differentiator/2(e), Sliding differentiator1/1(e)
  Integrator1/1 -> Sum/2

== system CAMFC2_04_Quad_03_R2017b/Agent #4/Decenteralized Cooperaive Controller #4/Cooperative Position Controller #4/Differentiator2 ==
  x_d : Inport
  Integrator : Integrator  InitialCondition=zeros(N+1,n0)
  Integrator1 : Integrator  InitialCondition=zeros(N+1,n0)
  Sliding differentiator : MATLAB Function  TreatAsAtomicUnit=on
  Sliding differentiator1 : MATLAB Function  TreatAsAtomicUnit=on
  Sum : Sum  Inputs=|-+
  Dx_d : Outport
  wires:
  Integrator1/1 -> Sum/2
  Sum/1 -> Sliding differentiator1/1(e), Sliding differentiator/2(e)
  x_d/1 -> Sum/1
  Integrator/1 -> Sliding differentiator/1(u1)
  Sliding differentiator1/1(Du1) -> Integrator/1
  Sliding differentiator/1(u) -> Dx_d/1, Integrator1/1

== system CAMFC2_04_Quad_03_R2017b/Agent #4/Decenteralized Cooperaive Controller #4/Rotational AMFC #4/Differentiator ==
  x_d : Inport
  Integrator : Integrator  InitialCondition=zeros(n,1)
  Integrator1 : Integrator  InitialCondition=zeros(n,1)
  Sliding differentiator : MATLAB Function  TreatAsAtomicUnit=on
  Sliding differentiator1 : MATLAB Function  TreatAsAtomicUnit=on
  Sum : Sum  Inputs=|-+
  Dx_d : Outport
  wires:
  Integrator1/1 -> Sum/2
  Sum/1 -> Sliding differentiator1/1(e), Sliding differentiator/2(e)
  x_d/1 -> Sum/1
  Integrator/1 -> Sliding differentiator/1(u1)
  Sliding differentiator1/1(Du1) -> Integrator/1
  Sliding differentiator/1(u) -> Dx_d/1, Integrator1/1

== system CAMFC2_04_Quad_03_R2017b/Agent #4/Decenteralized Cooperaive Controller #4/Velocity AMFC #4/Differentiator ==
  x_d : Inport
  Integrator : Integrator  InitialCondition=zeros(n0,1)
  Integrator1 : Integrator  InitialCondition=zeros(n0,1)
  Sliding differentiator : MATLAB Function  TreatAsAtomicUnit=on
  Sliding differentiator1 : MATLAB Function  TreatAsAtomicUnit=on
  Sum : Sum  Inputs=|-+
  Dx_d : Outport
  wires:
  Integrator1/1 -> Sum/2
  Sum/1 -> Sliding differentiator1/1(e), Sliding differentiator/2(e)
  x_d/1 -> Sum/1
  Integrator/1 -> Sliding differentiator/1(u1)
  Sliding differentiator1/1(Du1) -> Integrator/1
  Sliding differentiator/1(u) -> Dx_d/1, Integrator1/1

== system CAMFC2_04_Quad_03_R2017b/Agent #1/Decenteralized Cooperaive Controller #1/Cooperative Position Controller #1/DRE1/P1 ==
  a1 : Inport
  Agent_Num : Inport  Port=2
  DLE1 : MATLAB Function  TreatAsAtomicUnit=on
  DRE2 : MATLAB Function  TreatAsAtomicUnit=on
  Gain : Gain  Gain=-1
  Integrator1 : Integrator
  State_Num : Constant
  p1 : Outport
  wires:
  Gain/1 -> Integrator1/1
  Integrator1/1 -> DRE2/4(val_exp)
  DRE2/1(p) -> p1/1
  a1/1 -> DLE1/1(a_hat), DRE2/3(a_hat)
  DLE1/1(b) -> Gain/1
  Agent_Num/1 -> DLE1/2(Agent_Num), DRE2/1(Agent_Num)
  State_Num/1 -> DLE1/3(State_Num), DRE2/2(State_Num)

== system CAMFC2_04_Quad_03_R2017b/Agent #1/Decenteralized Cooperaive Controller #1/Cooperative Position Controller #1/DRE1/P2 ==
  a2 : Inport
  Agent_Num : Inport  Port=2
  DLE1 : MATLAB Function  TreatAsAtomicUnit=on
  DRE2 : MATLAB Function  TreatAsAtomicUnit=on
  Gain : Gain  Gain=-1
  Integrator1 : Integrator
  State_Num : Constant  Value=2
  p2 : Outport
  wires:
  State_Num/1 -> DRE2/2(State_Num), DLE1/3(State_Num)
  Agent_Num/1 -> DRE2/1(Agent_Num), DLE1/2(Agent_Num)
  DLE1/1(b) -> Gain/1
  a2/1 -> DRE2/3(a_hat), DLE1/1(a_hat)
  DRE2/1(p) -> p2/1
  Integrator1/1 -> DRE2/4(val_exp)
  Gain/1 -> Integrator1/1

== system CAMFC2_04_Quad_03_R2017b/Agent #1/Decenteralized Cooperaive Controller #1/Cooperative Position Controller #1/DRE1/P3 ==
  a3 : Inport
  Agent_Num : Inport  Port=2
  DLE1 : MATLAB Function  TreatAsAtomicUnit=on
  DRE2 : MATLAB Function  TreatAsAtomicUnit=on
  Gain : Gain  Gain=-1
  Integrator1 : Integrator
  State_Num : Constant  Value=3
  p3 : Outport
  wires:
  Gain/1 -> Integrator1/1
  Integrator1/1 -> DRE2/4(val_exp)
  DRE2/1(p) -> p3/1
  a3/1 -> DLE1/1(a_hat), DRE2/3(a_hat)
  DLE1/1(b) -> Gain/1
  Agent_Num/1 -> DLE1/2(Agent_Num), DRE2/1(Agent_Num)
  State_Num/1 -> DLE1/3(State_Num), DRE2/2(State_Num)

== system CAMFC2_04_Quad_03_R2017b/Agent #2/Decenteralized Cooperaive Controller #2/Cooperative Position Controller #2/DRE2/P1 ==
  a1 : Inport
  Agent_Num : Inport  Port=2
  DLE1 : MATLAB Function  TreatAsAtomicUnit=on
  DRE2 : MATLAB Function  TreatAsAtomicUnit=on
  Gain : Gain  Gain=-1
  Integrator1 : Integrator
  State_Num : Constant
  p1 : Outport
  wires:
  State_Num/1 -> DRE2/2(State_Num), DLE1/3(State_Num)
  Agent_Num/1 -> DRE2/1(Agent_Num), DLE1/2(Agent_Num)
  DLE1/1(b) -> Gain/1
  a1/1 -> DRE2/3(a_hat), DLE1/1(a_hat)
  DRE2/1(p) -> p1/1
  Integrator1/1 -> DRE2/4(val_exp)
  Gain/1 -> Integrator1/1

== system CAMFC2_04_Quad_03_R2017b/Agent #2/Decenteralized Cooperaive Controller #2/Cooperative Position Controller #2/DRE2/P2 ==
  a2 : Inport
  Agent_Num : Inport  Port=2
  DLE1 : MATLAB Function  TreatAsAtomicUnit=on
  DRE2 : MATLAB Function  TreatAsAtomicUnit=on
  Gain : Gain  Gain=-1
  Integrator1 : Integrator
  State_Num : Constant  Value=2
  p2 : Outport
  wires:
  Gain/1 -> Integrator1/1
  Integrator1/1 -> DRE2/4(val_exp)
  DRE2/1(p) -> p2/1
  a2/1 -> DLE1/1(a_hat), DRE2/3(a_hat)
  DLE1/1(b) -> Gain/1
  Agent_Num/1 -> DLE1/2(Agent_Num), DRE2/1(Agent_Num)
  State_Num/1 -> DLE1/3(State_Num), DRE2/2(State_Num)

== system CAMFC2_04_Quad_03_R2017b/Agent #2/Decenteralized Cooperaive Controller #2/Cooperative Position Controller #2/DRE2/P3 ==
  a3 : Inport
  Agent_Num : Inport  Port=2
  DLE1 : MATLAB Function  TreatAsAtomicUnit=on
  DRE2 : MATLAB Function  TreatAsAtomicUnit=on
  Gain : Gain  Gain=-1
  Integrator1 : Integrator
  State_Num : Constant  Value=3
  p3 : Outport
  wires:
  State_Num/1 -> DRE2/2(State_Num), DLE1/3(State_Num)
  Agent_Num/1 -> DRE2/1(Agent_Num), DLE1/2(Agent_Num)
  DLE1/1(b) -> Gain/1
  a3/1 -> DRE2/3(a_hat), DLE1/1(a_hat)
  DRE2/1(p) -> p3/1
  Integrator1/1 -> DRE2/4(val_exp)
  Gain/1 -> Integrator1/1

== system CAMFC2_04_Quad_03_R2017b/Agent #3/Decenteralized Cooperaive Controller #3/Cooperative Position Controller #3/DRE3/P1 ==
  a1 : Inport
  Agent_Num : Inport  Port=2
  DLE1 : MATLAB Function  TreatAsAtomicUnit=on
  DRE2 : MATLAB Function  TreatAsAtomicUnit=on
  Gain : Gain  Gain=-1
  Integrator1 : Integrator
  State_Num : Constant
  p1 : Outport
  wires:
  Gain/1 -> Integrator1/1
  Integrator1/1 -> DRE2/4(val_exp)
  DRE2/1(p) -> p1/1
  a1/1 -> DLE1/1(a_hat), DRE2/3(a_hat)
  DLE1/1(b) -> Gain/1
  Agent_Num/1 -> DLE1/2(Agent_Num), DRE2/1(Agent_Num)
  State_Num/1 -> DLE1/3(State_Num), DRE2/2(State_Num)

== system CAMFC2_04_Quad_03_R2017b/Agent #3/Decenteralized Cooperaive Controller #3/Cooperative Position Controller #3/DRE3/P2 ==
  a2 : Inport
  Agent_Num : Inport  Port=2
  DLE1 : MATLAB Function  TreatAsAtomicUnit=on
  DRE2 : MATLAB Function  TreatAsAtomicUnit=on
  Gain : Gain  Gain=-1
  Integrator1 : Integrator
  State_Num : Constant  Value=2
  p2 : Outport
  wires:
  State_Num/1 -> DRE2/2(State_Num), DLE1/3(State_Num)
  Agent_Num/1 -> DRE2/1(Agent_Num), DLE1/2(Agent_Num)
  DLE1/1(b) -> Gain/1
  a2/1 -> DRE2/3(a_hat), DLE1/1(a_hat)
  DRE2/1(p) -> p2/1
  Integrator1/1 -> DRE2/4(val_exp)
  Gain/1 -> Integrator1/1

== system CAMFC2_04_Quad_03_R2017b/Agent #3/Decenteralized Cooperaive Controller #3/Cooperative Position Controller #3/DRE3/P3 ==
  a3 : Inport
  Agent_Num : Inport  Port=2
  DLE1 : MATLAB Function  TreatAsAtomicUnit=on
  DRE2 : MATLAB Function  TreatAsAtomicUnit=on
  Gain : Gain  Gain=-1
  Integrator1 : Integrator
  State_Num : Constant  Value=3
  p3 : Outport
  wires:
  Gain/1 -> Integrator1/1
  Integrator1/1 -> DRE2/4(val_exp)
  DRE2/1(p) -> p3/1
  a3/1 -> DLE1/1(a_hat), DRE2/3(a_hat)
  DLE1/1(b) -> Gain/1
  Agent_Num/1 -> DLE1/2(Agent_Num), DRE2/1(Agent_Num)
  State_Num/1 -> DLE1/3(State_Num), DRE2/2(State_Num)

== system CAMFC2_04_Quad_03_R2017b/Agent #4/Decenteralized Cooperaive Controller #4/Cooperative Position Controller #4/DRE4/P1 ==
  a1 : Inport
  Agent_Num : Inport  Port=2
  DLE1 : MATLAB Function  TreatAsAtomicUnit=on
  DRE2 : MATLAB Function  TreatAsAtomicUnit=on
  Gain : Gain  Gain=-1
  Integrator1 : Integrator
  State_Num : Constant
  p1 : Outport
  wires:
  State_Num/1 -> DRE2/2(State_Num), DLE1/3(State_Num)
  Agent_Num/1 -> DRE2/1(Agent_Num), DLE1/2(Agent_Num)
  DLE1/1(b) -> Gain/1
  a1/1 -> DRE2/3(a_hat), DLE1/1(a_hat)
  DRE2/1(p) -> p1/1
  Integrator1/1 -> DRE2/4(val_exp)
  Gain/1 -> Integrator1/1

== system CAMFC2_04_Quad_03_R2017b/Agent #4/Decenteralized Cooperaive Controller #4/Cooperative Position Controller #4/DRE4/P2 ==
  a2 : Inport
  Agent_Num : Inport  Port=2
  DLE1 : MATLAB Function  TreatAsAtomicUnit=on
  DRE2 : MATLAB Function  TreatAsAtomicUnit=on
  Gain : Gain  Gain=-1
  Integrator1 : Integrator
  State_Num : Constant  Value=2
  p2 : Outport
  wires:
  Gain/1 -> Integrator1/1
  Integrator1/1 -> DRE2/4(val_exp)
  DRE2/1(p) -> p2/1
  a2/1 -> DLE1/1(a_hat), DRE2/3(a_hat)
  DLE1/1(b) -> Gain/1
  Agent_Num/1 -> DLE1/2(Agent_Num), DRE2/1(Agent_Num)
  State_Num/1 -> DLE1/3(State_Num), DRE2/2(State_Num)

== system CAMFC2_04_Quad_03_R2017b/Agent #4/Decenteralized Cooperaive Controller #4/Cooperative Position Controller #4/DRE4/P3 ==
  a3 : Inport
  Agent_Num : Inport  Port=2
  DLE1 : MATLAB Function  TreatAsAtomicUnit=on
  DRE2 : MATLAB Function  TreatAsAtomicUnit=on
  Gain : Gain  Gain=-1
  Integrator1 : Integrator
  State_Num : Constant  Value=3
  p3 : Outport
  wires:
  State_Num/1 -> DRE2/2(State_Num), DLE1/3(State_Num)
  Agent_Num/1 -> DRE2/1(Agent_Num), DLE1/2(Agent_Num)
  DLE1/1(b) -> Gain/1
  a3/1 -> DRE2/3(a_hat), DLE1/1(a_hat)
  DRE2/1(p) -> p3/1
  Integrator1/1 -> DRE2/4(val_exp)
  Gain/1 -> Integrator1/1

== matlab function CAMFC2_04_Quad_03_R2017b/Agent #1/Decenteralized Cooperaive Controller #1/Controller to Motors #1 ==
  data: u output; uT input; uR input
function u = fcn(uT,uR)

y1 = uR(4);
y2 = uR(5);
y3 = uR(6);

Y = [uT;y1;y2;y3];

u = Y;

end

== matlab function CAMFC2_04_Quad_03_R2017b/Agent #1/Decenteralized Cooperaive Controller #1/Cooperative Position Controller #1/Adaptive Law A#1 ==
  data: Agent_Num input; P input; A_hat input; gama2 parameter; rho2 parameter; T_i input; e input; DA_hat output; H parameter; N parameter; x0_hat_i input; P_struct parameter; n0 parameter
function DA_hat = fcn(Agent_Num,P,A_hat,gama2,rho2,T_i,e,H,N,x0_hat_i,P_struct,n0)

%% 
c_i = T_i(1,:)' - T_i(Agent_Num+1,:)' - x0_hat_i;

%%
vA_hat = diag(A_hat);

P_struct(1).data = P.p1;
P_struct(2).data = P.p2;
P_struct(3).data = P.p3;
P_struct(4).data = P.p4;

Sum = zeros(n0,1);
for i=1:N  
    Sum = Sum + (H(Agent_Num,i) * P_struct(i).data * e((i-1)*n0+1:(i*n0),1)); %Adaptive law
end
    
DvA_hat = +gama2*diag(c_i)*Sum - (rho2*gama2*vA_hat);

DA_hat = diag(DvA_hat);

end

== matlab function CAMFC2_04_Quad_03_R2017b/Agent #1/Decenteralized Cooperaive Controller #1/Cooperative Position Controller #1/Adaptive Law g#1 ==
  data: Agent_Num input; g_hat input; gama1 parameter; rho1 parameter; P input; P_struct parameter; Dg_hat output; e input; H parameter; N parameter; n0 parameter
function Dg_hat = fcn(Agent_Num,g_hat,gama1,rho1,P,P_struct,e,H,N,n0)

P_struct(1).data = P.p1;
P_struct(2).data = P.p2;
P_struct(3).data = P.p3;
P_struct(4).data = P.p4;

Sum = zeros(n0,1);
for i=1:N  
    Sum = Sum + (H(Agent_Num,i) * P_struct(i).data * e((i-1)*n0+1:(i*n0),1)); %Adaptive law
end
    
Dg_hat = -gama1*Sum - (rho1*gama1*g_hat);

end

== matlab function CAMFC2_04_Quad_03_R2017b/Agent #1/Decenteralized Cooperaive Controller #1/Cooperative Position Controller #1/DRE1/MATLAB Function1 ==
  data: inp input; otp output
function otp = fcn(inp)

otp = diag(inp);

end

== matlab function CAMFC2_04_Quad_03_R2017b/Agent #1/Decenteralized Cooperaive Controller #1/Cooperative Position Controller #1/DRE1/P1/DLE1 ==
  data: a_hat input; b output; Agent_Num input; State_Num input; H parameter; Q parameter
function b = fcn(a_hat,Agent_Num,State_Num, H, Q)

h = H(Agent_Num,Agent_Num);
q = Q(State_Num,State_Num);
Delta = (a_hat^2) + (2*q*h);
b = 2*sqrt(Delta);

end

== matlab function CAMFC2_04_Quad_03_R2017b/Agent #1/Decenteralized Cooperaive Controller #1/Cooperative Position Controller #1/DRE1/P1/DRE2 ==
  data: Agent_Num input; State_Num input; a_hat input; p output; val_exp input; H parameter; Q parameter
function p = fcn(Agent_Num,State_Num,a_hat,val_exp,H, Q)

p_init = 1;
h = H(Agent_Num,Agent_Num);
q = Q(State_Num,State_Num);
Delta = (a_hat^2) + (2*q*h);
p0 = (1/h) * (a_hat - sqrt(Delta));
w0 = 1 / (p_init - p0);
b = 2*sqrt(Delta);
w = (h/b) + (w0 - (h/b))*exp(val_exp);
p = p0 + (1/w);

end

== matlab function CAMFC2_04_Quad_03_R2017b/Agent #2/Decenteralized Cooperaive Controller #2/Controller Interpreter #2 ==
  data: ut_i input; uT_i output; PHI_d_i output
function [uT_i,PHI_d_i] = fcn(ut_i)

%%
f0 = sqrt((ut_i(1)^2)+(ut_i(2)^2)+(ut_i(3)^2));
psi_d = 0;
phi_d = asin( min(max(((sin(psi_d)*ut_i(1) - cos(psi_d)*ut_i(2)) / (f0+1e-3)),-1),1) );
theta_d = atan( (cos(psi_d)*ut_i(1) + sin(psi_d)*ut_i(2)) / (ut_i(3)+1e-3) );
PHI_d_i = [phi_d;theta_d;psi_d]; 
uT_i = f0;

end

== matlab function CAMFC2_04_Quad_03_R2017b/Agent #2/Decenteralized Cooperaive Controller #2/Controller to Motors #2 ==
  data: u output; uT input; uR input
function u = fcn(uT,uR)

y1 = uR(4);
y2 = uR(5);
y3 = uR(6);

Y = [uT;y1;y2;y3];

u = Y;

end

== matlab function CAMFC2_04_Quad_03_R2017b/Agent #1/Decenteralized Cooperaive Controller #1/Cooperative Position Controller #1/Differentiator0/Sliding differentiator1 ==
  data: Du1 output; e input; k2 parameter; alpha parameter
function Du1 = fcn(e,k2,alpha)

a=k2;

ABS = abs(e);
SGN = e ./ (ABS + alpha);
Du1 = - a*SGN;

end

== matlab function CAMFC2_04_Quad_03_R2017b/Agent #2/Decenteralized Cooperaive Controller #2/Cooperative Position Controller #2/Adaptive Law A#2 ==
  data: Agent_Num input; P input; A_hat input; gama2 parameter; rho2 parameter; T_i input; e input; DA_hat output; H parameter; N parameter; x0_hat_i input; P_struct parameter; n0 parameter
function DA_hat = fcn(Agent_Num,P,A_hat,gama2,rho2,T_i,e,H,N,x0_hat_i,P_struct,n0)

%% 
c_i = T_i(1,:)' - T_i(Agent_Num+1,:)' - x0_hat_i;

%%
vA_hat = diag(A_hat);

P_struct(1).data = P.p1;
P_struct(2).data = P.p2;
P_struct(3).data = P.p3;
P_struct(4).data = P.p4;

Sum = zeros(n0,1);
for i=1:N  
    Sum = Sum + (H(Agent_Num,i) * P_struct(i).data * e((i-1)*n0+1:(i*n0),1)); %Adaptive law
end
    
DvA_hat = +gama2*diag(c_i)*Sum - (rho2*gama2*vA_hat);

DA_hat = diag(DvA_hat);

end

== matlab function CAMFC2_04_Quad_03_R2017b/Agent #2/Decenteralized Cooperaive Controller #2/Cooperative Position Controller #2/Adaptive Law g#2 ==
  data: Agent_Num input; g_hat input; gama1 parameter; rho1 parameter; P input; P_struct parameter; Dg_hat output; e input; H parameter; N parameter; n0 parameter
function Dg_hat = fcn(Agent_Num,g_hat,gama1,rho1,P,P_struct,e,H,N,n0)

P_struct(1).data = P.p1;
P_struct(2).data = P.p2;
P_struct(3).data = P.p3;
P_struct(4).data = P.p4;

Sum = zeros(n0,1);
for i=1:N  
    Sum = Sum + (H(Agent_Num,i) * P_struct(i).data * e((i-1)*n0+1:(i*n0),1)); %Adaptive law
end
    
Dg_hat = -gama1*Sum - (rho1*gama1*g_hat);

end

== matlab function CAMFC2_04_Quad_03_R2017b/Agent #1/Decenteralized Cooperaive Controller #1/Cooperative Position Controller #1/Differentiator0/Sliding differentiator ==
  data: u output; u1 input; e input; k1 parameter; alpha parameter
function u = fcn(u1,e,k1,alpha)

b=k1;

ABS = abs(e);
SGN = e ./ (ABS + alpha);
u = u1 - b*((ABS.^0.5).*SGN); 

end

== matlab function CAMFC2_04_Quad_03_R2017b/Agent #1/Decenteralized Cooperaive Controller #1/Cooperative Position Controller #1/DRE1/MATLAB Function ==
  data: inp input; otp output
function otp = fcn(inp)

otp = diag(inp);

end

== matlab function CAMFC2_04_Quad_03_R2017b/Agent #1/Plant #1/MATLAB Function ==
  data: XT_V input; XR input; U input; t input; DP output; Dv output; Kd parameter; Ka parameter; M parameter; J parameter; ge parameter; DXR output; noise_amp parameter; noise_frq parameter
function [DP,Dv,DXR] = fcn(XT_V,XR,U,t,Kd,Ka,M,J,ge,noise_amp, noise_frq)

phi = XR(1);
theta = XR(2);
psi = XR(3);

Rq = [cos(psi)*cos(theta) -sin(psi)*cos(phi)+cos(psi)*sin(theta)*sin(phi) sin(psi)*sin(phi)+cos(psi)*sin(theta)*cos(phi);
    sin(psi)*cos(theta) cos(psi)*cos(phi)+sin(psi)*sin(theta)*sin(phi) -cos(psi)*sin(phi)+sin(psi)*sin(theta)*cos(phi);
    -sin(theta) cos(theta)*sin(phi) cos(theta)*cos(phi)]; 

R_omega = [1 0 -sin(theta);
    0 cos(phi) cos(theta)*sin(phi);
    0 -sin(phi) cos(theta)*cos(phi)];

EXT_PRD = External_Product3(XR(4:6),(J*XR(4:6)));

FTT = Rq * [0;0;U(1)];
TTT = U(2:4);

DP = XT_V;
DPHI = (R_omega)^(-1) * XR(4:6); 
Dv = (1/M)*(FTT - Kd*XT_V - M*M*[0;0;ge]) + Rq*(noise_amp*sin(noise_frq*t))*[0;0;1]; 
Dw = (J^(-1))*(TTT - Ka*XR(4:6) - EXT_PRD) + (noise_amp*sin(noise_frq*t)*[1;1;1]);
DXR = [DPHI;Dw];

end

== matlab function CAMFC2_04_Quad_03_R2017b/Agent #2/Decenteralized Cooperaive Controller #2/Cooperative Position Controller #2/DRE2/MATLAB Function ==
  data: inp input; otp output
function otp = fcn(inp)

otp = diag(inp);

end

== matlab function CAMFC2_04_Quad_03_R2017b/Agent #2/Decenteralized Cooperaive Controller #2/Cooperative Position Controller #2/DRE2/MATLAB Function1 ==
  data: inp input; otp output
function otp = fcn(inp)

otp = diag(inp);

end

== matlab function CAMFC2_04_Quad_03_R2017b/Agent #2/Decenteralized Cooperaive Controller #2/Cooperative Position Controller #2/DRE2/P1/DLE1 ==
  data: a_hat input; b output; Agent_Num input; State_Num input; H parameter; Q parameter
function b = fcn(a_hat,Agent_Num,State_Num, H, Q)

h = H(Agent_Num,Agent_Num);
q = Q(State_Num,State_Num);
Delta = (a_hat^2) + (2*q*h);
b = 2*sqrt(Delta);

end

== matlab function CAMFC2_04_Quad_03_R2017b/Agent #2/Decenteralized Cooperaive Controller #2/Cooperative Position Controller #2/DRE2/P1/DRE2 ==
  data: Agent_Num input; State_Num input; a_hat input; p output; val_exp input; H parameter; Q parameter
function p = fcn(Agent_Num,State_Num,a_hat,val_exp,H, Q)

p_init = 1;
h = H(Agent_Num,Agent_Num);
q = Q(State_Num,State_Num);
Delta = (a_hat^2) + (2*q*h);
p0 = (1/h) * (a_hat - sqrt(Delta));
w0 = 1 / (p_init - p0);
b = 2*sqrt(Delta);
w = (h/b) + (w0 - (h/b))*exp(val_exp);
p = p0 + (1/w);

end
